simulink model "jointTorqController_reachPosStep"  (Simulink 8.0)
settings: Solver=FixedStepDiscrete  StartTime=0.0  StopTime=Inf  FixedStep=Ts  RelTol=1e-3
values from neighbouring files (symbols this model uses):
  dqiRef = 10*pi/180    (= 0.174532925199)    [init_jointTorqController_reachPos.m]
  GRAV_COMP = 1    [init_jointTorqController_reachPos.m]
  Kd = 2*sqrt(Kp)*0.01*diag([ones(1,4),ones(1,4),myK*ones(1,6),myK*ones(1,6)])    [init_jointTorqController_reachPos.m]
  KdOnOff = 1    [init_jointTorqController_reachPos.m]
  Kp = diag([KpArms,KpArms,KpLegs,KpLegs])    [init_jointTorqController_reachPos.m]
  KpOnOff = 1    [init_jointTorqController_reachPos.m]
  qErr = 1*pi/180    (= 0.0174532925199)    [init_jointTorqController_reachPos.m]
  qjDes = zeros(ROBOT_DOF,1)    [init_jointTorqController_reachPos.m]
  refMask = zeros(ROBOT_DOF,1)    [init_jointTorqController_reachPos.m]
  refMaskGravComp = zeros(ROBOT_DOF,1)    [init_jointTorqController_reachPos.m]
  ROBOT_DOF = 20    [init_jointTorqController_reachPos.m]
  Ts = 0.01    [init_jointTorqController_reachPos.m]
libraries: WBCLibrary x12
settings Model: Creator=nunoguedelha  LastModifiedBy=nunoguedelha

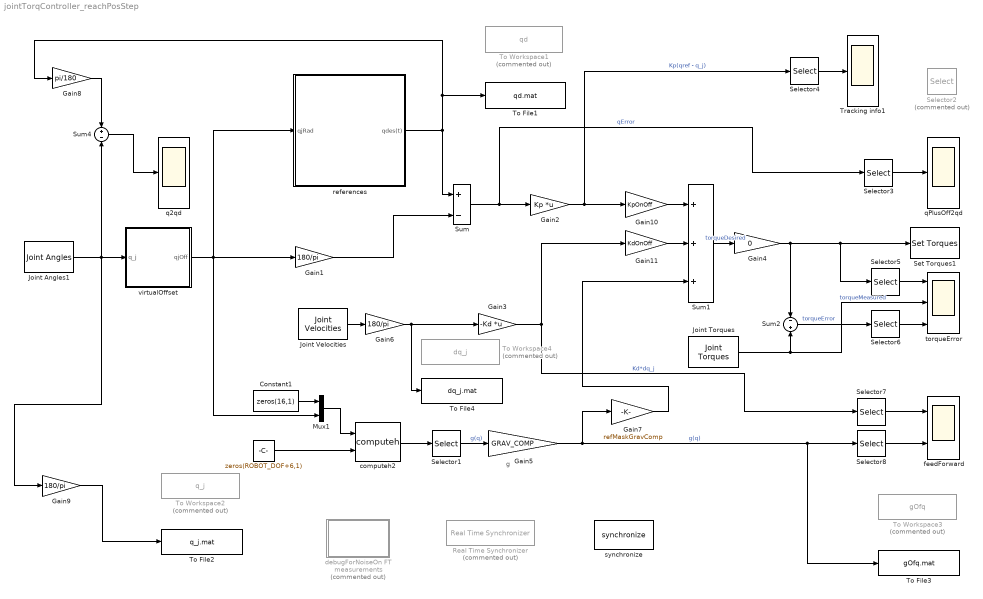
== system jointTorqController_reachPosStep ==
  note: g
  " " : Constant  Tag=bla  Value=zeros(ROBOT_DOF+6,1)  SampleTime=-1
  Constant1 : Constant  Value=zeros(16,1)  SampleTime=-1
  Gain1 : Gain  Gain=180/pi
  Gain10 : Gain  Gain=KpOnOff
  Gain11 : Gain  Gain=KdOnOff
  Gain2 : Gain  Gain=Kp  Multiplication=Matrix(K*u)
  Gain3 : Gain  Gain=-Kd  Multiplication=Matrix(K*u)
  Gain4 : Gain  Gain=0
  Gain5 : Gain  Gain=GRAV_COMP
  Gain6 : Gain  Gain=180/pi
  Gain7 : Gain  Gain=refMaskGravComp
  Gain8 : Gain  Gain=pi/180
  Gain9 : Gain  Gain=180/pi
  Joint Angles1 : WBCLibrary/wholeBodyStates/Joint Angles  robotName=robotName  localName=localName
  Joint Torques : WBCLibrary/wholeBodyStates/Joint Torques  robotName=robotName  localName=localName
  Joint Velocities : WBCLibrary/wholeBodyStates/Joint Velocities  robotName=robotName  localName=localName
  Mux1 : Mux  Inputs=2
  Real Time Synchronizer : WBCLibrary/Utilities/Real Time Synchronizer  Priority=-10  Commented=on  threadPeriod=Ts
  Selector1 : Selector  InputPortWidth=ROBOT_DOF+6  IndexOptions=Index vector (dialog)  Indices=[7:ROBOT_DOF+6]  OutputSizes=1
  Selector2 : Selector  Commented=on  InputPortWidth=2*ROBOT_DOF  IndexOptions=Index vector (dialog)  Indices=[19 (ROBOT_DOF+19)]  OutputSizes=1
  Selector{3..8} (6 alike) : Selector  InputPortWidth=ROBOT_DOF  IndexOptions=Index vector (dialog)  Indices=displayMask  OutputSizes=1
  Set Torques1 : WBCLibrary/wholeBodyActuators/Set Torques  val=6  robotName=robotName  localName=localName
  Sum : Sum  Inputs=+-
  Sum1 : Sum  Inputs=+++
  Sum2 : Sum  Inputs=-|+
  Sum4 : Sum  Inputs=+|-
  To File1 : ToFile  Filename=qd.mat  SaveFormat=Timeseries
  To File2 : ToFile  Filename=q_j.mat  SaveFormat=Timeseries
  To File3 : ToFile  Filename=gOfq.mat  SaveFormat=Timeseries
  To File4 : ToFile  Filename=dq_j.mat  SaveFormat=Timeseries
  To Workspace1 : ToWorkspace  Commented=on  VariableName=qd  SampleTime=-1  SaveFormat=Timeseries
  To Workspace2 : ToWorkspace  Commented=on  VariableName=q_j  SampleTime=-1  SaveFormat=Timeseries
  To Workspace3 : ToWorkspace  Commented=on  VariableName=gOfq  SampleTime=-1  SaveFormat=Timeseries
  To Workspace4 : ToWorkspace  Commented=on  VariableName=dq_j  SampleTime=-1  SaveFormat=Timeseries
  Tracking info1 : Scope
      settings: ShowLegends=on  TimeRange=20  YMin=-60  YMax=80  SaveName=ScopeData6
  computeh2 : WBCLibrary/wholeBodyModel/Dynamics/computeh  val=7  robotname=robotName  localname=localName
  debugForNoiseOn FT measurements : Subsystem  Commented=on
  feedForward : Scope  NumInputPorts=2
      settings: ShowLegends=on  TimeRange=70  YMin=-6.5e-05~-1.4  YMax=1e-05~0.5
  q2qd : Scope
      settings: ShowLegends=on  TimeRange=20  YMin=-60  YMax=80  SaveName=ScopeData7
  qPlusOff2qd : Scope
      settings: TickLabels=on  ShowLegends=on  TimeRange=20  YMin=-35  YMax=30  SaveName=ScopeData3
  references : Subsystem
  synchronize : WBCLibrary/Utilities/synchronize  rate=0.010  scaleFactor=1
  torqueError : Scope  NumInputPorts=3
      settings: ShowLegends=on  TimeRange=20  YMin=-1~-5e-05~-8.39912e-323  YMax=1~0.00075~8.39912e-323
  virtualOffset : MATLAB Function  TreatAsAtomicUnit=on
  wires:
  Gain1/1 -> Sum/2
  Sum/1 -> Gain2/1, Selector3/1  "qError"
  Gain2/1 -> Gain10/1, Selector4/1  "Kp(qref - q_j)"
  Joint Velocities/1 -> Gain6/1
  Gain3/1 -> Selector7/1, Gain11/1  "Kd*dq_j"
  Sum1/1 -> Gain4/1  "torqueDesired"
  computeh2/1 -> Selector1/1
  Mux1/1 -> computeh2/1
  Constant1/1 -> Mux1/1
  Selector1/1 -> Gain5/1  "g(q)"
  Joint Torques/1 -> torqueError/2, Sum2/2  "torqueMeasured"
  Sum2/1 -> Selector6/1  "torqueError"
  Gain5/1 -> Gain7/1, To File3/1, Selector8/1  "g(q)"
  Gain6/1 -> To File4/1, Gain3/1
  " "/1 -> computeh2/2
  Gain4/1 -> Sum2/1, Selector5/1, Set Torques1/1
  Selector3/1 -> qPlusOff2qd/1
  Selector4/1 -> Tracking info1/1
  Gain7/1 -> Sum1/3
  virtualOffset/1(qjOff) -> references/1(qjRad), Gain1/1, Mux1/2
  Sum4/1 -> q2qd/1
  Gain8/1 -> Sum4/1
  references/1(qdes(t)) -> Sum/1, To File1/1, Gain8/1
  Joint Angles1/1 -> Gain9/1, Sum4/2, virtualOffset/1(q_j)
  Gain9/1 -> To File2/1
  Gain10/1 -> Sum1/1
  Gain11/1 -> Sum1/2
  Selector5/1 -> torqueError/1
  Selector6/1 -> torqueError/3
  Selector7/1 -> feedForward/1
  Selector8/1 -> feedForward/2

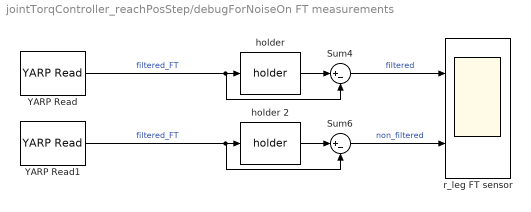
== system jointTorqController_reachPosStep/debugForNoiseOn FT measurements ==
  Sum4 : Sum  Inputs=|+-
  Sum6 : Sum  Inputs=|+-
  YARP Read : WBCLibrary/Utilities/YARP Read  portName='/wholeBodyDynamicsTree/filtered/r_leg_ft_sensor:o'  signalSize=6  blocking=off  timestamp=off  autoconnect=on  errorOnConnection=off
  YARP Read1 : WBCLibrary/Utilities/YARP Read  portName='/icub/right_leg/analog:o'  signalSize=6  blocking=off  timestamp=off  autoconnect=on  errorOnConnection=off
  "holder " : WBCLibrary/Utilities/holder 
  holder 2 : WBCLibrary/Utilities/holder 
  r_leg FT sensor : Scope  NumInputPorts=2
      settings: ShowLegends=on  TimeRange=10  YMin=-10~-15  YMax=15~20  SaveName=ScopeData5
  wires:
  "holder "/1 -> Sum4/1
  YARP Read/1 -> Sum4/2, "holder "/1  "filtered_FT"
  Sum6/1 -> r_leg FT sensor/2  "non_filtered"
  YARP Read1/1 -> Sum6/2, holder 2/1  "filtered_FT"
  holder 2/1 -> Sum6/1
  Sum4/1 -> r_leg FT sensor/1  "filtered"

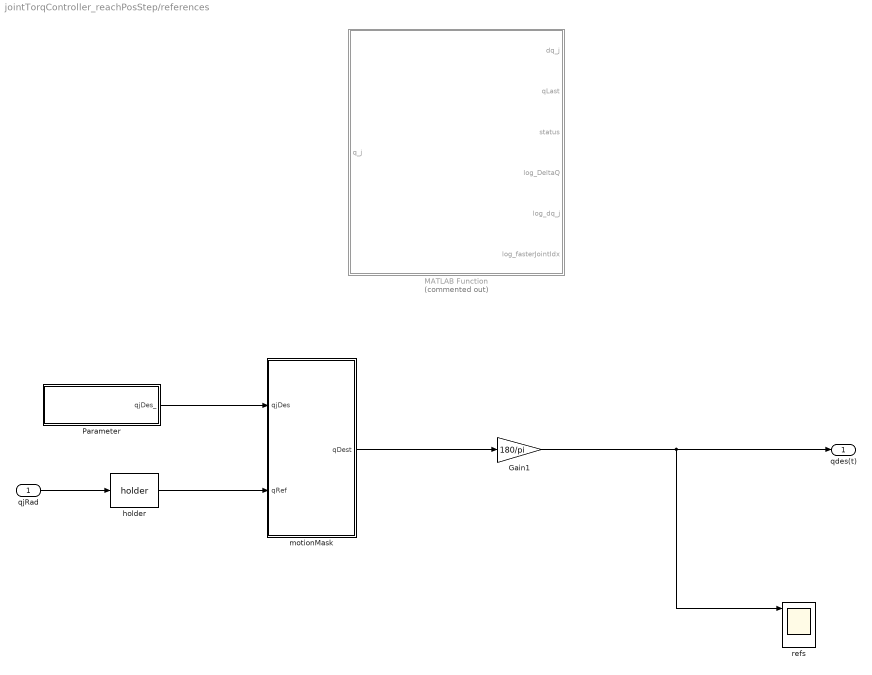
== system jointTorqController_reachPosStep/references ==
  qjRad : Inport
  Gain1 : Gain  Gain=180/pi
  MATLAB Function : MATLAB Function  Commented=on  TreatAsAtomicUnit=on
  Parameter : MATLAB Function  TreatAsAtomicUnit=on
  "holder " : WBCLibrary/Utilities/holder 
  motionMask : MATLAB Function  TreatAsAtomicUnit=on
  refs : Scope  NumInputPorts=3
      settings: ShowLegends=on  TimeRange=70  YMin=-40~-32.5~-30  YMax=140~0~10  SaveName=ScopeData2
  qdes(t) : Outport
  wires:
  qjRad/1 -> "holder "/1
  "holder "/1 -> motionMask/2(qRef)
  motionMask/1(qDest) -> Gain1/1
  Gain1/1 -> qdes(t)/1, refs/1
  Parameter/1(qjDes_) -> motionMask/1(qjDes)

== matlab function references/MATLAB Function ==
  data: dq_j output double; qjDes parameter double; dqiRef parameter double; q_j input double; ROBOT_DOF parameter double; qErr parameter double; Ts parameter double; qLast output double; status output double; log_DeltaQ output double; log_dq_j output double; log_fasterJointIdx output double
function [dq_j, qLast, status, log_DeltaQ, log_dq_j, log_fasterJointIdx]  = checkStopCond(qjDes, dqiRef, q_j, ROBOT_DOF, qErr, Ts)
%#codegen

% define the maximum speed (in degrees) of the reference revolute single joint
% (single DOF). This is done manually:
% joints rotation speed is considered constant, so we only get centripete 
% acceleration . $|a_n| = \frac{v^2}{R} = R dq^2$
% => $dqiRef = \sqrt{\frac{|a_n|}{R}}$
% As a_n max should not exceed 1/10 g,
% $dqiRef = \sqrt{\frac{1}{R}} ~ sqrt(1/0.4) ~ 1.5 rad.s^{-1} = 85 degs.s^{-1}$ for $g ~
% 10m.s^{-2}$.
% Let's have a margin and define $45 deg.s^{-1}$ (signed value)
persistent fasterJointIdx;
persistent last_dq_j;
persistent last_deltaQ;
persistent stopMotionVec;
persistent state;

dq_j = zeros(ROBOT_DOF,1);

%% handle state
if isempty(state)
    state = 0;
end

% update positions relative to the destination
DeltaQ = qjDes - q_j;

% Fill static variables
if isempty(last_deltaQ)
    last_deltaQ = DeltaQ;
end

if isempty(stopMotionVec)
    stopMotionVec = ones(ROBOT_DOF,1);
end

if isempty(fasterJointIdx)
    % Select joint for which rotation will have the highest speed.
    % This shall be the high boundary speed for all joints. We shall set this
    % boundary to the maximum speed 'dqiRef' required for neglecting the angular
    % and linear acceleration to be measured by the sensors, w.r.t. the gravity
    % measurements.
    [~,idx_of_max] = max(abs(DeltaQ));
    fasterJointIdx = uint8(idx_of_max); % convert to uint8
end

if isempty(last_dq_j)
    last_dq_j = zeros(ROBOT_DOF,1);
end


if state == 0
    %% Program joint velocity for current timeslot

    % If angles are small, avoid computing dq_j, just use same velocities for
    % all joints.
    if abs(DeltaQ(fasterJointIdx))>(5*pi/180)
        dq_j = DeltaQ*(dqiRef/abs(DeltaQ(fasterJointIdx)));
        last_dq_j = dq_j;
    else
        dq_j = last_dq_j;
    end
    
    % We shall stop as soon as the joint closest to its respective end position
    % reaches the end position vicinity (d<0.1 deg) or overshoots.
    % Considering that the velocity or position tracking accuracy is not perfect, 
    % we should monitor each joint independently.
    for i = 1:ROBOT_DOF
    if abs(DeltaQ(i))<(dqiRef*10*Ts) ... % proximity
            || last_deltaQ(i)*DeltaQ(i)<0 % overshoot
        % mark respective joint for stopping
        stopMotionVec(i) = 0;
    end
    end
    
    % Stop the joints that reached destination
    dq_j = dq_j.*stopMotionVec;
    
    if any(dq_j)
        state = 0;
        last_deltaQ = DeltaQ;
    else
        % final configuration reached
        state = 1;
    end
end

% save last position
qLast = q_j;
% output state
status = state;

%log DeltaQ and dq_j
log_DeltaQ = DeltaQ;
log_dq_j = dq_j;
log_fasterJointIdx = fasterJointIdx;

% we would clear the static variables here but 'clear' is not supported
% in generated code

end

== matlab function references/motionMask ==
  data: qjDes input double; qRef input double; refMask parameter double; qDest output double; ROBOT_DOF parameter double
function qDest = motionMask(qjDes,qRef,refMask,ROBOT_DOF)
%#codegen

% Target position
qDest = qjDes.*refMask + qRef.*(ones(ROBOT_DOF,1)-refMask);

== matlab function references/Parameter ==
  data: qjDes parameter double; qjDes_ output double
function qjDes_ = getParameter(qjDes)
%#codegen
qjDes_ = qjDes;

== matlab function virtualOffset ==
  data: q_j input double; qjOff output double; randOffsets parameter double
function qjOff = virtualOffset(q_j,randOffsets)
%#codegen


qjOff = q_j + randOffsets;
